simulink model "demo_01_whole_model"  (R2016b)
settings: Solver=FixedStepDiscrete  StartTime=0.0  StopTime=10.0  FixedStep=50e-6  RelTol=1e-3
settings Model: Creator=anony  LastModifiedBy=anony

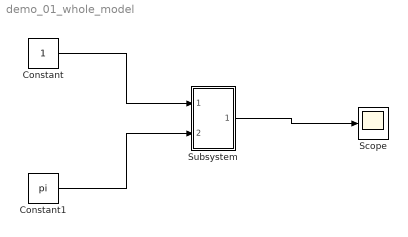
== system demo_01_whole_model ==
  Constant : Constant
  Constant1 : Constant  Value=pi
  Scope : Scope
  Subsystem : Subsystem
  wires:
  Constant/1 -> Subsystem/1(In1)
  Constant1/1 -> Subsystem/2(In2)
  Subsystem/1(Out1) -> Scope/1

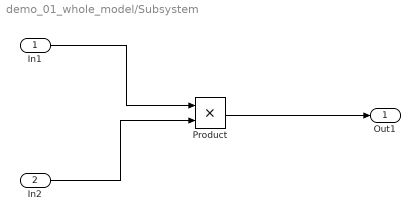
== system demo_01_whole_model/Subsystem ==
  In1 : Inport
  In2 : Inport  Port=2
  Product : Product
  Out1 : Outport
  wires:
  In2/1 -> Product/2
  In1/1 -> Product/1
  Product/1 -> Out1/1
